simulink model "FullyConnectedMMG"  (R2020b)
settings: Solver=ode3  StartTime=0.0  StopTime=TimeS  FixedStep=Ts  RelTol=1e-3
values from neighbouring files (symbols this model uses):
  fr = 60    [MMG_Parameters.m]
  Lgs = 600e-6    (= 0.0006)    [MMG_Parameters.m]
  MaxWind = 18    [MMG_Parameters.m]
  MicroVol = 575    [MMG_Parameters.m]
  MinWind = 3    [MMG_Parameters.m]
  NomVol = 600    [MMG_Parameters.m]
  NomWind = 10    [MMG_Parameters.m]
  Pnombb = 400    [MMG_Parameters.m]
  PnomDG = 150e3    (= 150000)    [MMG_Parameters.m]
  PnomWT = 400e3    (= 400000)    [MMG_Parameters.m]
  Rgs = 20e-6    (= 2e-05)    [MMG_Parameters.m]
  RtCapM1 = (5.1)*1e-1    (= 0.51)    [MMG_Parameters.m]
  RtCapM2 = (5.1)*1e-1    (= 0.51)    [MMG_Parameters.m]
  SOC = [70,80,75,65]    [MMG_Parameters.m]
  Ts = 8e-4    (= 0.0008)    [MMG_Parameters.m]    (also in SolveMONO.m = 0.005)
  Vgrid = 25e3    (= 25000)    [MMG_Parameters.m]
  VMic = 575    [MMG_Parameters.m]
  Vs = 120e3    (= 120000)    [MMG_Parameters.m]
undefined symbols (not defined in the file or in its folder): DiscIntNeverNeededParam
libraries: powerlib x64, simulink x24, powerlib_meascontrol x16
(part 2 of 5)

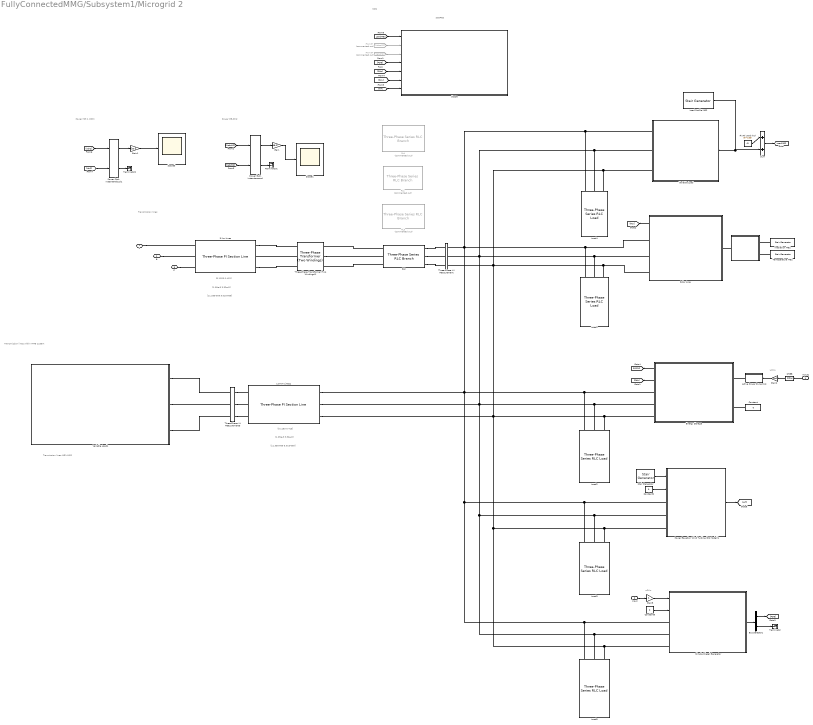
== system FullyConnectedMMG/Subsystem1/Microgrid 2 ==
  note: [0.1153 0.413]
  note: SCOPES
  note: w2Kw
  note: w2Kw
  note: MG2
  note: Transmission lines
  note: Power MG-Grid
  note: [0.1153 0.413]
  note: Transmission lines within MMG system
  note: [11.33e-009 5.01e-009]
  note: Tranmission lines MG1-MG2
  note: [1.05e-3 3.32e-3]
  note: [1.05e-3 3.32e-3]
  note: [11.33e-009 5.01e-009]
  note: Power MG 2 -MGm
  Input1 : Inport
  Input : Inport  Port=2
  " " : Subsystem  VariantControl=T6NotZero  mask{Pvr=200, Dfac=0.98, Tfac=0.3, Tsc=25}
      mask prompts: Pvr "Rated Power (kW)"; Dfac "Derating Factor"; Tfac "Temperature Factor"; Tsc "Standard Temperature (C)"
  1.5 Km Lines1 : powerlib/Elements/Three-Phase PI Section Line  LConnTagsString=a|b|c  RConnTagsString=A|B|C  Length=1.5  Frequency=fr  Resistances=[0.1153 1.413]  Inductances=[1.05e-3 3.32e-3]  Capacitances=[11.33e-009 5.01e-009]
  3 Km Lines : powerlib/Elements/Three-Phase PI Section Line  LConnTagsString=a|b|c  RConnTagsString=A|B|C  Length=3.5  Frequency=fr  Resistances=[0.0153 0.213]  Inductances=[1.05e-3 3.32e-3]  Capacitances=[11.33e-009 5.01e-009]
  Active Power Dynamics : Subsystem  VariantControl=T6NotZero
      mask Display: disp('1 / (1 + s T_P)','texmode','on');
  Bus Selector1 : BusSelector  OutputSignals=Active power P (W),Reactive power Q (var)
  Constant : Constant  Value=0
  Constant2 : Constant  Value=0
  Constant5 : Constant  Value=0
  Energy Storage : Subsystem  mask(Grid-connected Energy Storage (PQ Model)){Vn=NomVol, Fn=60, PnomkW=Pnombb, kWh_Rated=RtCapM2, Efficiency=96, LimitVec=[90 10], RechargeSOC=11, Precharge=50, autoRecharge=off, Initial_kWh_pc=SOC(2), PQvec=[500e3 0]}
      mask prompts: Vn "Nominal L-L Voltage [Vrms]"; Fn "Nominal Frequency [Hz]"; PnomkW "Rated Power [kW]"; kWh_Rated "Rated Capacity [kWh]"; Efficiency "Overall System Efficiency [%]"; LimitVec "Upper/Lower Charge Limits [%]"; RechargeSOC "SOC to Recharge [%]"; Precharge "Recharge Rate [% of Rated Power]"; autoRecharge "Enable Auto-Recharge"; Initial_kWh_pc "Initial State-of-Charge [0-100%]"; PQvec "Initial Active/Reactive Cmds"
      mask help:
      | The energy storage block models a generic grid-connected energy storage system (ESS), most commonly a battery system. This is a system-level model that does not contain any power electronics, but is useful for load flow, phasor, and hybrid phasor-EMT simulations. The inputs to this block are the commanded active and reactive power of the ESS. The ESS is assumed to have four quadrent operation.
      |
      | For more detailed ESS models, consider the battery block in the Drives library. Consider using this PQ Model to perform load flow studies and switch to a more detailed model when full EMT studies or more advanced controls are required.
      |
      | Note: The initial active/reactive power commands must be specified for use for Load Flow analysis.
      mask init: same as FullyConnectedMMG/Subsystem1/Microgrid 1/Energy Storage
      mask DialogControl Container7 Prompt: Grid Connection Properties
      mask DialogControl Container11 Prompt: Charge/Discharge Controls
      mask DialogControl Container12 Prompt: Initial Conditions
      mask Display: image(imread('Battery.png'))
  Fixed Load (Kw) : Constant  Value=(3)*(1e3)  VectorParams1D=off
  From34 : From  Commented=on  GotoTag=IabcM2  TagVisibility=global
      settings: CloseFcn=tagdialog Close
  From37 : From  Commented=on  GotoTag=VabcM2  TagVisibility=global
      settings: CloseFcn=tagdialog Close
  Gain : Gain  Gain=1e-3
  Gain1 : Gain  Gain=1e-3
  Gain2 : Gain  Gain=1e0
  Gain5 : Gain
  Irradiation MG2 : powerlib_meascontrol/Pulse & Signal Generators/Stair Generator  t=Time  e=IrMG2  Ts=Ts
  Load Profile MG2 : powerlib_meascontrol/Pulse & Signal Generators/Stair Generator  t=Time  e=PLoad2  Ts=Ts
  Load{1..5} (5 alike) : powerlib/Elements/Three-Phase Series RLC Load  LConnTagsString=A|B|C  Configuration=Y (grounded)  NominalVoltage=575  Vabc=[1e3 1e3 1e3]  Vabcp=[1e3 1e3 1e3]  NominalFrequency=60  UnbalancedPower=off  ActivePower=1e3  InductivePower=0  CapacitivePower=0  Pabc=[10e3 9e3 11e3]  QLabc=[100 90 110]  QCabc=[100 90 110]  Pabcp=[10e3 9e3 11e3]  QLabcp=[100 90 110]  QCabcp=[100 90 110]  Measurements=None  LoadType=constant Z
      settings: AttributesFormatString=P = %<ActivePower> W
  "Power (3ph, Instantaneous)" : powerlib_meascontrol/Measurements/Power (3ph, Instantaneous)
  "Power (3ph, Instantaneous)1" : powerlib_meascontrol/Measurements/Power (3ph, Instantaneous)
  Power Equation Wind Turbine (PQ Model)1 : Subsystem  AncestorBlock=|  mask{Unom=NomWind, Umax=MaxWind, Umin=MinWind, Pselect=Simple Cubic Power, rp=5, Cp=16/27, rho=1.225, Pnom=PnomWT, Uvec=[1:1:30], Pvec=1e-1*[0,0,0,0,21359.3750000000,58193.5000000000,104316.125000000,157104.500000000,213935.875000000,272187.500000000,329236.625000000,382460.500000000,429236.375000000,466941.500000000,492953.125000000,500000,500000,500000,500000,500000,500000,500000,500000,500000,500000,0,0,0,0,0], Tp=0.1, Tq=1, ReactP=30}
      | exampleMicrogridLibrary/Power Equation
      | Wind Turbine
      | (PQ Model)
      mask prompts: Unom "Nominal Wind Speed [m/s]"; Umax "Maximum Operating Wind [m/s]"; Umin "Minimum Operating Wind [m/s]"; Pselect "Wind Turbine Power Method"; rp "Blade Radius, r [m]"; Cp "Performance Coefficient, Cp"; rho "Air Density, rho [kg/m^3]"; Pnom "Nominal Power, [W]"; Uvec "Wind Vec [m/s]"; Pvec "Power Vec [W]"; Tp "Active Power Dynamics, Tp [s]"; Tq "Reactive Power Dynamics, Tq [s]"; ReactP "Reactive Power Percentage [%]"
      mask help:
      | Simple Wind Turbine that serves as an Active and Reactive Power Source depending on the Wind Power Curve.
      |
      | The Wind Turbine Power Curve can be defined by:
      | - Dimentions of the wind turbine
      | - Simple cubic power curve
      | - Look-up vector from a wind turbine data sheet.
      mask init:
      | A = pi*rp^2;
      | 
      | if Pselect == 1,
      |     Pmax = 1/2*rho*Cp*A*Umax^3;
      | elseif Pselect == 2,
      |     Pmax = Pnom;
      | else
      |     Pmax = max(Pvec);
      | end
      | Qmax = ReactP/100*Pmax;
      mask TypeOptions Pselect: Using Properties | Simple Cubic Power | Look-up Fit
      mask DialogControl Container4 Prompt: General
      mask DialogControl Container9 Prompt: Dimensions
      mask DialogControl Container12 Prompt: Cubic
      mask DialogControl Container7 Prompt: Lookup
      mask DialogControl Container8 Prompt: Dynamics
      mask Display:
      | image(imread('eolienne.bmp'))
      | 
      | color('white')
      | port_label('LConn',1,'A')
      | port_label('LConn',2,'B')
      | port_label('LConn',3,'C')
      | 
      | color('blue')
      | port_label('output',1,'m')
      | port_label('input',1,'Wind (m/s)')
      | port_label('input',2,'Qref')
  RL1 : powerlib/Elements/Three-Phase Series RLC Branch  Commented=on  LConnTagsString=A|B|C  RConnTagsString=A|B|C  BranchType=RL  Resistance=Rgs  Inductance=Lgs  Capacitance=inf  Measurements=None
  RL2 : powerlib/Elements/Three-Phase Series RLC Branch  LConnTagsString=A|B|C  RConnTagsString=A|B|C  BranchType=RL  Resistance=Rgs  Inductance=70e-6  Capacitance=inf  Measurements=None
  RL3 : powerlib/Elements/Three-Phase Series RLC Branch  Commented=on  LConnTagsString=A|B|C  RConnTagsString=A|B|C  BranchType=RL  Resistance=Rgs  Inductance=Lgs  Capacitance=inf  Measurements=None
  RL4 : powerlib/Elements/Three-Phase Series RLC Branch  Commented=on  LConnTagsString=A|B|C  RConnTagsString=A|B|C  BranchType=RL  Resistance=Rgs  Inductance=Lgs  Capacitance=inf  Measurements=None
  Scope : Subsystem
  Scope1 : Scope
  Scope3 : Scope
  Simple Diesel Generator : Subsystem  AncestorBlock=|  mask{Pn=PnomDG, Vn=VMic, Fn=fr, Tp=0.1, Tq=1, ReactP=30, Ts=Ts}
      | exampleMicrogridLibrary/Power Equation
      | Wind Turbine
      | (PQ Model)
      mask prompts: Pn "Generator Rated Power [W]"; Vn "Rated Voltage [V]"; Fn "Rated Frequency [Hz]"; Tp "Active Power Dynamics, Tp [s]"; Tq "Reactive Power Dynamics, Tq [s]"; ReactP "Reactive Power Percentage [%]"; Ts "Sample Time"
      mask help:
      | Simple Wind Turbine that serves as an Active and Reactive Power Source depending on the Wind Power Curve.
      |
      | The Wind Turbine Power Curve can be defined by:
      | - Dimentions of the wind turbine
      | - Simple cubic power curve
      | - Look-up vector from a wind turbine data sheet.
      mask init:
      | Pmax = 320e3;
      | Qmax = ReactP/100*Pmax;
      mask DialogControl Container4 Prompt: General
      mask DialogControl Container8 Prompt: Dynamics
      mask Display:
      | image(imread('DGEN.jpg'));
      | color('black')
  Solar Array : Subsystem  mask(Grid-Connected PV Array (PQ Model)){Vn=MicroVol, Fn=fr, P0=500e3}
      mask prompts: Vn "Nominal L-L Voltage [Vrms]"; Fn "Nominal Frequency [Hz]"; P0 "Initial Power [W]"
      mask help:
      | This block models a grid-connected solar array using the Three-Phase Dynamic Load block. This is a system-level model that does not contain any power electronics, but is useful for load flow, phasor, and hybrid phasor-EMT simulations. The input to this block is the power output of the grid connected PV array, not irradiance.
      |
      | For more detailed PV models, consider the PV Array block in the Renewables library. Consider using this PQ Model to perform load flow studies and switch to a more detailed model when full EMT studies are required.
      |
      | Note: The array power must be specified for use for Load Flow analysis.
      mask init:
      | % P0 = Irr0*TotalArea*Efficiency/100;
      | P0 = -P0;
      mask Display:
      | image(imread('PV_Farm.jpg'))
      | color('white')
      | port_label('input',1,'P')
      | port_label('output',1,'m')
      | port_label('Rconn',1,'A')
      | port_label('Rconn',2,'B')
      | port_label('Rconn',3,'C')
  Stair Generator : powerlib_meascontrol/Pulse & Signal Generators/Stair Generator  t=Time  e=WindM2  Ts=Ts
  Sum : Sum  Inputs=|++
  Temeperature MG2 : powerlib_meascontrol/Pulse & Signal Generators/Stair Generator  t=Time  e=TempMG2  Ts=Ts
  Terminator : Terminator
  Terminator1 : Terminator
  Terminator2 : Terminator
  Three-Phase Transformer (Two Windings)1 : powerlib/Elements/Three-Phase Transformer (Two Windings)  Winding1Connection=Yg  Winding2Connection=Yg  CoreType=Three single-phase transformers  SetSaturation=off  Hysteresis=off  DataFile='hysteresis'  SetInitialFlux=off  Measurements=None  UNITS=pu  NominalPower=[ 25e6 , 60 ]  Winding1=[575 , 0.002 , 0.08 ]  Winding2=[575 , 0.002 , 0.08 ]  Rm=500  Lm=500  L0=0.5  Saturation=[ 0,0 ; 0.0024,1.2 ; 1.0,1.52 ]  InitialFluxes=[ 0.8 , -0.8 , 0.7 ]  BreakLoop=off  DiscreteSolver=Trapezoidal iterative  DataType=off  TransfoNumber=1
  Three-Phase V-I Measurement : powerlib/Measurements/Three-Phase V-I Measurement  VoltageMeasurement=phase-to-ground  SetLabelV=on  LabelV=VabcM2  Vpu=off  VpuLL=off  CurrentMeasurement=yes  SetLabelI=on  LabelI=IabcM2  Ipu=off  Pbase=100e6  Vbase=500e3  OutputType=Complex  PhasorSimulation=off  PSBequivalent=0
  Three-Phase V-I Measurement3 : powerlib/Measurements/Three-Phase V-I Measurement  VoltageMeasurement=phase-to-ground  SetLabelV=on  LabelV=Vsh2  Vpu=off  VpuLL=off  CurrentMeasurement=yes  SetLabelI=on  LabelI=Ish2  Ipu=off  Pbase=100e6  Vbase=500e3  OutputType=Complex  PhasorSimulation=off  PSBequivalent=0
  Variable Load : Subsystem  mask(Variable Load (PQ Model)){Vn=MicroVol, Fn=fr, PF=1, Load0=20e3}
      mask prompts: Vn "Nominal L-L Voltage [Vrms]"; Fn "Nominal Frequency [Hz]"; PF "Power Factor [0 to 1]"; Load0 "Initial Load [W]"
      mask help:
      | The Variable Load block is a lumped approximation for a distribution feeder. For non-unity power factor loads, the input (active power) is scaled accordingly to generate a desired load.
      |
      | Note: The initial input load must be specified for use for Load Flow analysis.
      mask init:
      | P0 = Load0;
      | Q0 = Load0*sqrt(1/PF-1);
      mask Display:
      | image(imread('Residential.jpg'))
      | color('white')
      | port_label('input',1,'Load')
      | port_label('Rconn',1,'A')
      | port_label('Rconn',2,'B')
      | port_label('Rconn',3,'C')
  Variable Load1 : Subsystem  mask(Variable Load (PQ Model)){Vn=MicroVol, Fn=fr, PF=1, Load0=20e3}
      mask prompts: Vn "Nominal L-L Voltage [Vrms]"; Fn "Nominal Frequency [Hz]"; PF "Power Factor [0 to 1]"; Load0 "Initial Load [W]"
      mask help:
      | The Variable Load block is a lumped approximation for a distribution feeder. For non-unity power factor loads, the input (active power) is scaled accordingly to generate a desired load.
      |
      | Note: The initial input load must be specified for use for Load Flow analysis.
      mask init:
      | P0 = Load0;
      | Q0 = Load0*sqrt(1/PF-1);
      mask Display:
      | image(imread('Sharing.jpg'))
      | color('black')
      | % port_label('input',1,'Load')
      | port_label('Rconn',1,'A')
      | port_label('Rconn',2,'B')
      | port_label('Rconn',3,'C')
  ZHBB : ZeroOrderHold  SampleTime=Ts
  A : PMIOPort  Side=Left
  B : PMIOPort  Port=2  Side=Left
  C : PMIOPort  Port=3  Side=Left
  tag scope: LoadMG2=global, SOCM2=global
  wires:
  Sum/1 -> [LoadMG2]
  Solar Array/1(m) -> [Ppv]
  Load Profile MG2/1 -> Sum/2, Variable Load/1(Load)
  Fixed Load (Kw)/1 -> Sum/1
  Power Equation Wind Turbine (PQ Model)1/1(m) -> [WT]
  Constant2/1 -> Power Equation Wind Turbine (PQ Model)1/2(Qref (pu))
  Gain2/1 -> Active Power Dynamics/1(In)
  " "/1(PowerOut) -> Solar Array/1(P)
  Gain5/1 -> Simple Diesel Generator/1(Pref (pu))
  Bus Selector1/1 -> [PDG]  "<Active power P (W)>"
  Bus Selector1/2 -> Terminator/1  "<Reactive power Q (var)>"
  Constant5/1 -> Simple Diesel Generator/2(Qref (pu))
  Simple Diesel Generator/1(m) -> Bus Selector1/1
  Input1/1 -> ZHBB/1
  ZHBB/1 -> Gain2/1
  Input/1 -> Gain5/1
  Stair Generator/1 -> Power Equation Wind Turbine (PQ Model)1/1(Wind (m/s))
  Irradiation MG2/1 -> " "/1(Irra)
  Temeperature MG2/1 -> " "/2(Temp)
  Energy Storage/2(Pbatt) -> [Pbb]
  Constant/1 -> Energy Storage/2(Qref)
  Active Power Dynamics/1(Out) -> Energy Storage/1(Pref)
  [LoadMG2] -> Scope/1(LOAD)  "Load M2"
  From37/1 -> Scope/2(VABC)
  From34/1 -> Scope/3(IABC)
  [PDG] -> Scope/4(PDG)
  [Pbb] -> Scope/5(PBB)
  [Ppv] -> Scope/6(PPV)
  [WT] -> Scope/7(PWT)
  Energy Storage/1(SOC (%)) -> [SOCM2]
  [VabcM2] -> "Power (3ph, Instantaneous)"/1
  "Power (3ph, Instantaneous)"/2 -> Terminator1/1
  Gain/1 -> Scope1/1
  "Power (3ph, Instantaneous)"/1 -> Gain/1
  [IabcM2] -> "Power (3ph, Instantaneous)"/2
  "Power (3ph, Instantaneous)1"/1 -> Gain1/1
  [Ish2] -> "Power (3ph, Instantaneous)1"/2
  "Power (3ph, Instantaneous)1"/2 -> Terminator2/1
  Gain1/1 -> Scope3/1
  [Vsh2] -> "Power (3ph, Instantaneous)1"/1
  connections:
  Three-Phase Transformer (Two Windings)1/LConn2 -- 3 Km Lines/LConn2
  3 Km Lines/LConn1 -- Three-Phase Transformer (Two Windings)1/LConn1
  3 Km Lines/LConn3 -- Three-Phase Transformer (Two Windings)1/LConn3
  A/RConn1 -- 3 Km Lines/RConn1
  B/RConn1 -- 3 Km Lines/RConn2
  C/RConn1 -- 3 Km Lines/RConn3
  RL2/RConn1 -- Three-Phase Transformer (Two Windings)1/RConn1
  RL2/RConn3 -- Three-Phase Transformer (Two Windings)1/RConn3
  Three-Phase Transformer (Two Windings)1/RConn2 -- RL2/RConn2
  Variable Load/RConn1 -- Load4/LConn1 -- 1.5 Km Lines1/LConn1 -- Load5/LConn1 -- Simple Diesel Generator/LConn1 -- Load3/LConn1 -- Power Equation Wind Turbine (PQ Model)1/LConn1 -- Energy Storage/RConn1 -- Load2/LConn1 -- Solar Array/RConn1 -- Load1/LConn1 -- Three-Phase V-I Measurement/RConn1
  Variable Load/RConn2 -- Load4/LConn2 -- 1.5 Km Lines1/LConn2 -- Load5/LConn2 -- Simple Diesel Generator/LConn2 -- Load3/LConn2 -- Power Equation Wind Turbine (PQ Model)1/LConn2 -- Energy Storage/RConn2 -- Load2/LConn2 -- Load1/LConn2 -- Solar Array/RConn2 -- Three-Phase V-I Measurement/RConn2
  Variable Load/RConn3 -- Load4/LConn3 -- 1.5 Km Lines1/LConn3 -- Load5/LConn3 -- Simple Diesel Generator/LConn3 -- Load3/LConn3 -- Power Equation Wind Turbine (PQ Model)1/LConn3 -- Energy Storage/RConn3 -- Load2/LConn3 -- Load1/LConn3 -- Solar Array/RConn3 -- Three-Phase V-I Measurement/RConn3
  Variable Load1/RConn3 -- Three-Phase V-I Measurement3/RConn3
  Variable Load1/RConn1 -- Three-Phase V-I Measurement3/RConn1
  Variable Load1/RConn2 -- Three-Phase V-I Measurement3/RConn2
  Three-Phase V-I Measurement3/LConn1 -- 1.5 Km Lines1/RConn1
  Three-Phase V-I Measurement3/LConn2 -- 1.5 Km Lines1/RConn2
  Three-Phase V-I Measurement3/LConn3 -- 1.5 Km Lines1/RConn3
  RL2/LConn2 -- Three-Phase V-I Measurement/LConn2
  RL2/LConn1 -- Three-Phase V-I Measurement/LConn1
  RL2/LConn3 -- Three-Phase V-I Measurement/LConn3

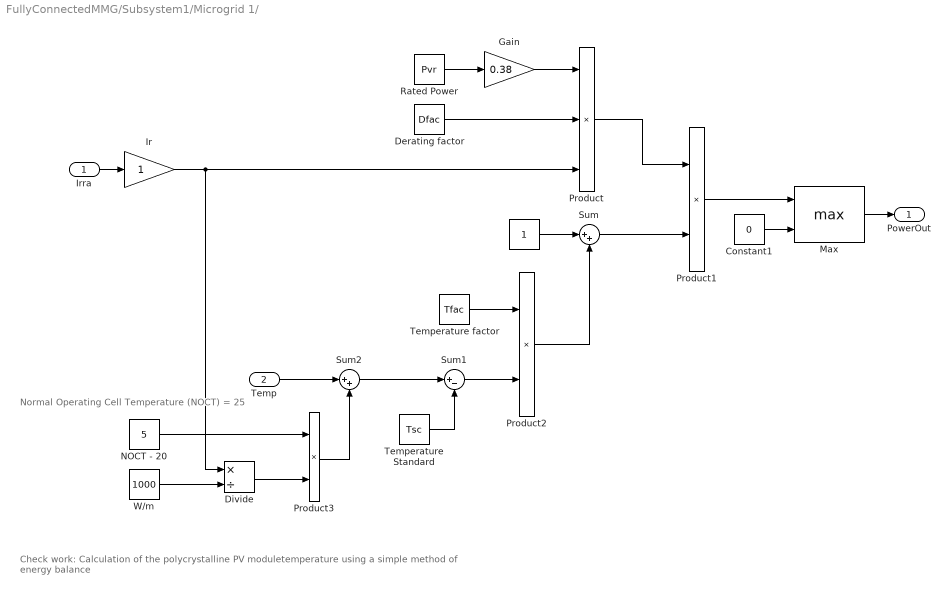
== system FullyConnectedMMG/Subsystem1/Microgrid 1/  ==
  note: Check work: Calculation of the polycrystalline PV moduletemperature using a simple method of energy balance
  note: Normal Operating Cell Temperature (NOCT) = 25
  Irra : Inport
  Temp : Inport  Port=2
  " " : Constant
  Constant1 : Constant  Value=0
  Derating factor : Constant  Value=Dfac
  Divide : Product  Inputs=*/
  Gain : Gain  Gain=0.38
  Ir : Gain
  Max : MinMax  Function=max  Inputs=2
  NOCT - 20 : Constant  Value=5
  Product : Product  Inputs=3
  Product1 : Product
  Product2 : Product
  Product3 : Product
  Rated Power : Constant  Value=Pvr
  Sum : Sum  Inputs=|++
  Sum1 : Sum  Inputs=|+-
  Sum2 : Sum  Inputs=|++
  Temperature Standard : Constant  Value=Tsc
  Temperature factor : Constant  Value=Tfac
  W/m : Constant  Value=1000
  PowerOut : Outport  VectorParamsAs1DForOutWhenUnconnected=off
  wires:
  Rated Power/1 -> Gain/1
  Gain/1 -> Product/1
  Derating factor/1 -> Product/2
  Irra/1 -> Ir/1
  Product/1 -> Product1/1
  " "/1 -> Sum/1
  Product2/1 -> Sum/2
  Temperature factor/1 -> Product2/1
  Sum/1 -> Product1/2
  Sum1/1 -> Product2/2
  Temperature Standard/1 -> Sum1/2
  Temp/1 -> Sum2/1
  Sum2/1 -> Sum1/1
  Product3/1 -> Sum2/2
  NOCT - 20/1 -> Product3/1
  Divide/1 -> Product3/2
  W/m/1 -> Divide/2
  Ir/1 -> Divide/1, Product/3
  Constant1/1 -> Max/2
  Max/1 -> PowerOut/1
  Product1/1 -> Max/1

== system FullyConnectedMMG/Subsystem1/Microgrid 1/Active Power Dynamics1 ==
  In : Inport
  1/Tp : Gain  Gain=1/0.004
  Integrator : Integrator
  Sum : Sum  Inputs=|+-
  Out : Outport  VectorParamsAs1DForOutWhenUnconnected=off
  wires:
  Integrator/1 -> Out/1, Sum/2
  In/1 -> Sum/1
  1/Tp/1 -> Integrator/1
  Sum/1 -> 1/Tp/1

== system FullyConnectedMMG/Subsystem1/Microgrid 1/Energy Storage ==
  Pref : Inport
  Qref : Inport  Port=2
  Charge Limits : Subsystem
  Mux1 : Mux  Inputs=2
  Power Limits : Saturate  UpperLimit=Pnom  LowerLimit=-Pnom
  Reactive Power Capability : Subsystem
  Simple Battery Inverter : powerlib/Elements/Three-Phase Dynamic Load  NominalVoltage=[Vn Fn]  ActiveReactivePowers=[-500000 -3.38813e-13]  PositiveSequence=[0.999844 -0.0038635]  ExternalControl=on  NpNq=[1.3 2]  TimeConstants="[0  0  0  0]"  MinimumVoltage=0.7  Tfilter=1e-2  LoadFlowParameters=[4,0,0,0,0]
      link override Model/Discrete 3-phase PLL: Ts=Ts
      link override Model/Mean (Variable Frequency): Ts=Ts
      link override Model/Mean (Variable Frequency)1: Ts=Ts
      settings: SourceProductBaseCode=PS
  Stored Energy Calculation (%) : Subsystem
  Terminator : Terminator
  Unary Minus : UnaryMinus
  A : PMIOPort  Side=Right
  B : PMIOPort  Port=2  Side=Right
  C : PMIOPort  Port=3  Side=Right
  SOC (%) : Outport  VectorParamsAs1DForOutWhenUnconnected=off
  Pbatt : Outport  Port=2  VectorParamsAs1DForOutWhenUnconnected=off
  wires:
  Charge Limits/2(Qbatt) -> Reactive Power Capability/2(Qin)
  Qref/1 -> Charge Limits/3(Qin)
  Power Limits/1 -> Charge Limits/2(Pin)
  Charge Limits/1(Pbatt) -> Reactive Power Capability/1(Pin), Unary Minus/1, Pbatt/1, Stored Energy Calculation (%)/1(Pin)  "Pbatt"
  Stored Energy Calculation (%)/1(SE%) -> SOC (%)/1, Charge Limits/1(SOC (%))  "SOC (%)"
  Pref/1 -> Power Limits/1
  Reactive Power Capability/1(Qout) -> Mux1/2, Stored Energy Calculation (%)/2(Qin)  "Qbatt"
  Simple Battery Inverter/1 -> Terminator/1
  Mux1/1 -> Simple Battery Inverter/1
  Unary Minus/1 -> Mux1/1
  connections:
  Simple Battery Inverter/LConn1 -- A/RConn1
  Simple Battery Inverter/LConn3 -- C/RConn1
  Simple Battery Inverter/LConn2 -- B/RConn1

== system FullyConnectedMMG/Subsystem1/Microgrid 1/Power Equation Wind Turbine (PQ Model) ==
  Wind (m/s) : Inport
  Qref (pu) : Inport  Port=2
  Active Power Dynamics : Subsystem  VariantControl=T6NotZero
      mask Display: disp('1 / (1 + s T_P)','texmode','on');
  Ground : powerlib/Elements/Ground  LConnTagsString=a
  Mux : Mux  Inputs=2
  Reactive Power Dynamics : Subsystem  VariantControl=T6NotZero
      mask Display: disp('1 / (1 + s T_Q)','texmode','on');
  Saturation : Saturate  UpperLimit=Qmax  LowerLimit=-Qmax
  Scope : Scope
  Shunt (Numerical Stability) : powerlib/Elements/Three-Phase Series RLC Branch  LConnTagsString=A|B|C  RConnTagsString=A|B|C  BranchType=R  Resistance=1e3  Inductance=1e-3  Capacitance=1e-6  Measurements=None
  Three-Phase Dynamic Load : powerlib/Elements/Three-Phase Dynamic Load  NominalVoltage=[575 60]  ActiveReactivePowers=[20e3 1e3]  PositiveSequence=[0.994 -11.8]  ExternalControl=on  NpNq=[1.3 2]  TimeConstants="[0  0  0  0]"  MinimumVoltage=0.7  Tfilter=1e-4  LoadFlowParameters=[4,0,0,0,0]
      link override Model/Discrete 3-phase PLL: Ts=Ts
      link override Model/Mean (Variable Frequency): Ts=Ts
      link override Model/Mean (Variable Frequency)1: Ts=Ts
      settings: SourceProductBaseCode=PS
  Unary Minus : UnaryMinus
  Wind Turbine Power Equation : Subsystem
  A : PMIOPort  Side=Left
  B : PMIOPort  Port=2  Side=Left
  C : PMIOPort  Port=3  Side=Left
  m : Outport  VectorParamsAs1DForOutWhenUnconnected=off
  wires:
  Qref (pu)/1 -> Saturation/1
  Saturation/1 -> Reactive Power Dynamics/1(In)
  Reactive Power Dynamics/1(Out) -> Mux/2
  Mux/1 -> Three-Phase Dynamic Load/1
  Wind Turbine Power Equation/1(Pwind) -> Active Power Dynamics/1(In)
  Wind (m/s)/1 -> Wind Turbine Power Equation/1(Wind (m/s))
  Three-Phase Dynamic Load/1 -> m/1
  Active Power Dynamics/1(Out) -> Unary Minus/1
  Unary Minus/1 -> Scope/1, Mux/1
  connections:
  Ground/LConn1 -- Shunt (Numerical Stability)/RConn1 -- Shunt (Numerical Stability)/RConn2 -- Shunt (Numerical Stability)/RConn3
  Three-Phase Dynamic Load/LConn1 -- Shunt (Numerical Stability)/LConn1 -- A/RConn1
  Three-Phase Dynamic Load/LConn3 -- Shunt (Numerical Stability)/LConn3 -- C/RConn1
  Three-Phase Dynamic Load/LConn2 -- Shunt (Numerical Stability)/LConn2 -- B/RConn1

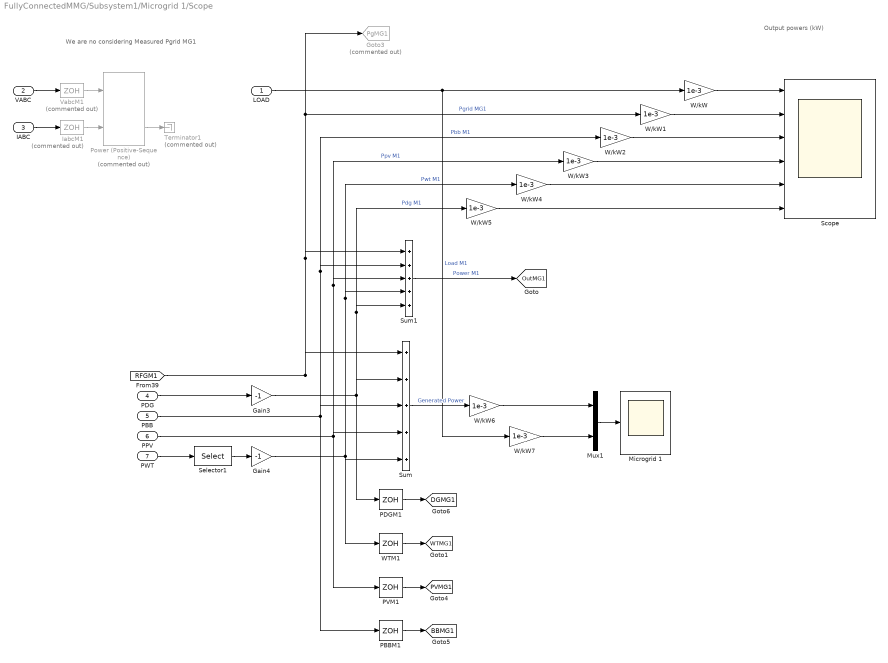
== system FullyConnectedMMG/Subsystem1/Microgrid 1/Scope ==
  note: Output powers (kW)
  note: We are no considering Measured Pgrid MG1
  LOAD : Inport
  VABC : Inport  Port=2
  IABC : Inport  Port=3
  PDG : Inport  Port=4
  PBB : Inport  Port=5
  PPV : Inport  Port=6
  PWT : Inport  Port=7
  Gain3 : Gain  Gain=-1
  Gain4 : Gain  Gain=-1
  Goto3 : Goto  Commented=on  GotoTag=PgMG1  TagVisibility=global
  IabcM1 : ZeroOrderHold  Commented=on  SampleTime=Ts
  Microgrid 1 : Scope
  Mux1 : Mux  Inputs=2
  PBBM1 : ZeroOrderHold  SampleTime=Ts
  PDGM1 : ZeroOrderHold  SampleTime=Ts
  PVM1 : ZeroOrderHold  SampleTime=Ts
  Power (Positive-Sequence) : powerlib_meascontrol/Measurements/Power (Positive-Sequence)  Commented=on  Freq=60  Vinit=[0, 0]  Iinit=[0, 0]  Ts=3e-4
      settings: SourceProductBaseCode=PS
  Scope : Scope  NumInputPorts=6
  Selector1 : Selector  InputPortWidth=3  IndexOptions=Index vector (dialog)  Indices=[2]  OutputSizes=1
  Sum : Sum  Inputs=|+++++
  Sum1 : Sum  Inputs=|+++++
  Terminator1 : Terminator  Commented=on
  VabcM1 : ZeroOrderHold  Commented=on  SampleTime=Ts
  W/kW{,1..7} (8 alike) : Gain  Gain=1e-3
  WTM1 : ZeroOrderHold  SampleTime=Ts
  tag scope: BBMG1=global, DGMG1=global, OutMG1=global, PVMG1=global, WTMG1=global
  wires:
  Power (Positive-Sequence)/2 -> Terminator1/1
  PPV/1 -> Sum/4, PVM1/1, Sum1/3, W/kW3/1  "Ppv M1"
  PBB/1 -> PBBM1/1, Sum/3, Sum1/2, W/kW2/1  "Pbb M1"
  [RFGM1] -> Sum1/1, Goto3/1, W/kW1/1, Sum/1  "Pgrid MG1"
  Mux1/1 -> Microgrid 1/1
  LOAD/1 -> W/kW7/1, W/kW/1  "Load M1"
  Gain4/1 -> WTM1/1, Sum/5, Sum1/4, W/kW4/1  "Pwt M1"
  PWT/1 -> Selector1/1
  Selector1/1 -> Gain4/1
  Sum1/1 -> [OutMG1]  "Power M1"
  Sum/1 -> W/kW6/1  "Generated Power"
  Gain3/1 -> PDGM1/1, Sum1/5, W/kW5/1, Sum/2  "Pdg M1"
  PDG/1 -> Gain3/1
  PDGM1/1 -> [DGMG1]
  PBBM1/1 -> [BBMG1]
  PVM1/1 -> [PVMG1]
  WTM1/1 -> [WTMG1]
  VabcM1/1 -> Power (Positive-Sequence)/1
  VABC/1 -> VabcM1/1
  IabcM1/1 -> Power (Positive-Sequence)/2
  IABC/1 -> IabcM1/1
  W/kW/1 -> Scope/1
  W/kW1/1 -> Scope/2
  W/kW2/1 -> Scope/3
  W/kW3/1 -> Scope/4
  W/kW4/1 -> Scope/5
  W/kW5/1 -> Scope/6
  W/kW6/1 -> Mux1/1
  W/kW7/1 -> Mux1/2

== system FullyConnectedMMG/Subsystem1/Microgrid 1/Simple Diesel Generator ==
  Pref (pu) : Inport
  Qref (pu) : Inport  Port=2
  Active Power Dynamics : Subsystem  VariantControl=T6NotZero
      mask Display: disp('1 / (1 + s T_P)','texmode','on');
  Ground : powerlib/Elements/Ground  LConnTagsString=a
  Mux : Mux  Inputs=2
  Reactive Power Dynamics : Subsystem  VariantControl=T6NotZero
      mask Display: disp('1 / (1 + s T_Q)','texmode','on');
  Saturation : Saturate  UpperLimit=Qmax  LowerLimit=-Qmax
  Shunt (Numerical Stability) : powerlib/Elements/Three-Phase Series RLC Branch  LConnTagsString=A|B|C  RConnTagsString=A|B|C  BranchType=R  Resistance=1e3  Inductance=1e-3  Capacitance=1e-6  Measurements=None
  Three-Phase Dynamic Load : powerlib/Elements/Three-Phase Dynamic Load  NominalVoltage=[Vn Fn]  ActiveReactivePowers=[20e3 1e3]  PositiveSequence=[0.994 -11.8]  ExternalControl=on  NpNq=[1.3 2]  TimeConstants="[0  0  0  0]"  MinimumVoltage=0.7  Tfilter=1e-4  LoadFlowParameters=[4,0,0,0,0]
      link override Model/Discrete 3-phase PLL: Ts=Ts
      link override Model/Discrete 3-phase PLL/Discrete PI Controller: Ts=Ts
      link override Model/Discrete 3-phase PLL/Discrete Rate Limiter: Ts=Ts
      link override Model/Discrete 3-phase PLL/Discrete Variable Frequency Mean value: Ts=Ts
      link override Model/Mean (Variable Frequency): Ts=Ts
      link override Model/Mean (Variable Frequency)1: Ts=Ts
      settings: SourceProductBaseCode=PS
  Unary Minus : UnaryMinus
  A : PMIOPort  Side=Left
  B : PMIOPort  Port=2  Side=Left
  C : PMIOPort  Port=3  Side=Left
  m : Outport  VectorParamsAs1DForOutWhenUnconnected=off
  wires:
  Pref (pu)/1 -> Active Power Dynamics/1(In)
  Mux/1 -> Three-Phase Dynamic Load/1
  Reactive Power Dynamics/1(Out) -> Mux/2
  Saturation/1 -> Reactive Power Dynamics/1(In)
  Qref (pu)/1 -> Saturation/1
  Three-Phase Dynamic Load/1 -> m/1
  Active Power Dynamics/1(Out) -> Unary Minus/1
  Unary Minus/1 -> Mux/1
  connections:
  B/RConn1 -- Shunt (Numerical Stability)/LConn2 -- Three-Phase Dynamic Load/LConn2
  C/RConn1 -- Shunt (Numerical Stability)/LConn3 -- Three-Phase Dynamic Load/LConn3
  A/RConn1 -- Shunt (Numerical Stability)/LConn1 -- Three-Phase Dynamic Load/LConn1
  Shunt (Numerical Stability)/RConn3 -- Shunt (Numerical Stability)/RConn2 -- Shunt (Numerical Stability)/RConn1 -- Ground/LConn1

== system FullyConnectedMMG/Subsystem1/Microgrid 1/Solar Array ==
  P : Inport
  Active Power Dynamics : Subsystem  VariantControl=T6NotZero
      mask Display: disp('1 / (1 + s T_P)','texmode','on');
  Bus Selector : BusSelector  OutputSignals=Active power P (W)
  Constant11 : Constant  Value=0
  Mux1 : Mux  Inputs=2
  Simple Solar Inverter : powerlib/Elements/Three-Phase Dynamic Load  NominalVoltage=[Vn Fn]  ActiveReactivePowers=[-250000 -3.38813e-13]  PositiveSequence=[0.999844 -0.0038635]  ExternalControl=on  NpNq=[1.3 2]  TimeConstants="[0  0  0  0]"  MinimumVoltage=0.7  Tfilter=1e-2  LoadFlowParameters=[4,0,0,0,0]
      link override Model/Discrete 3-phase PLL/Discrete PI Controller: Ts=Ts
      link override Model/Discrete 3-phase PLL/Discrete Rate Limiter: Ts=Ts
      link override Model/Discrete 3-phase PLL/Discrete Variable Frequency Mean value: Ts=Ts
      settings: SourceProductBaseCode=PS
  Unary Minus : UnaryMinus
  Unary Minus1 : UnaryMinus
  A : PMIOPort  Side=Right
  B : PMIOPort  Port=2  Side=Right
  C : PMIOPort  Port=3  Side=Right
  m : Outport  VectorParamsAs1DForOutWhenUnconnected=off
  wires:
  P/1 -> Active Power Dynamics/1(In)
  Unary Minus/1 -> Mux1/1
  Mux1/1 -> Simple Solar Inverter/1
  Constant11/1 -> Mux1/2
  Simple Solar Inverter/1 -> Bus Selector/1
  Bus Selector/1 -> Unary Minus1/1  "<Active power P (W)>"
  Unary Minus1/1 -> m/1
  Active Power Dynamics/1(Out) -> Unary Minus/1
  connections:
  Simple Solar Inverter/LConn2 -- B/RConn1
  Simple Solar Inverter/LConn3 -- C/RConn1
  Simple Solar Inverter/LConn1 -- A/RConn1

== system FullyConnectedMMG/Subsystem1/Microgrid 1/Variable Load ==
  Load : Inport
  Active Power Dynamics : Subsystem  VariantControl=T6NotZero
      mask Display: disp('1 / (1 + s T_P)','texmode','on');
  Dynamic Load Control : Subsystem
  Simple Three-Phase Load : powerlib/Elements/Three-Phase Dynamic Load  NominalVoltage=[Vn Fn]  ActiveReactivePowers=[200000 45883.1]  PositiveSequence=[0.999844 -0.0038635]  ExternalControl=on  NpNq=[1.3 2]  TimeConstants="[0  0  0  0]"  MinimumVoltage=0.7  Tfilter=1e-2  LoadFlowParameters=[4,0,0,0,0]
      link override Model/Discrete 3-phase PLL: Ts=Ts
      link override Model/Discrete 3-phase PLL/Discrete PI Controller: Ts=Ts
      link override Model/Discrete 3-phase PLL/Discrete Rate Limiter: Ts=Ts
      link override Model/Discrete 3-phase PLL/Discrete Variable Frequency Mean value: Ts=Ts
      link override Model/Discrete 3-phase PLL/Discrete  2nd-Order Filter: Ts=Ts
      link override Model/Mean (Variable Frequency): Ts=Ts
      link override Model/Mean (Variable Frequency)1: Ts=Ts
      settings: SourceProductBaseCode=PS
  Terminator : Terminator
  A : PMIOPort  Side=Right
  B : PMIOPort  Port=2  Side=Right
  C : PMIOPort  Port=3  Side=Right
  wires:
  Simple Three-Phase Load/1 -> Terminator/1
  Dynamic Load Control/1(PQ) -> Simple Three-Phase Load/1
  Load/1 -> Active Power Dynamics/1(In)
  Active Power Dynamics/1(Out) -> Dynamic Load Control/1(P0)
  connections:
  Simple Three-Phase Load/LConn1 -- A/RConn1
  Simple Three-Phase Load/LConn3 -- C/RConn1
  Simple Three-Phase Load/LConn2 -- B/RConn1

== system FullyConnectedMMG/Subsystem1/Microgrid 1/Variable Load1 ==
  Active Power Dynamics : Subsystem  VariantControl=T6NotZero
      mask Display: disp('1 / (1 + s T_P)','texmode','on');
  Dynamic Load Control : Subsystem
  Load2 : powerlib/Elements/Three-Phase Series RLC Load  LConnTagsString=A|B|C  Configuration=Y (grounded)  NominalVoltage=575  Vabc=[1e3 1e3 1e3]  Vabcp=[1e3 1e3 1e3]  NominalFrequency=60  UnbalancedPower=off  ActivePower=1e3  InductivePower=0  CapacitivePower=0  Pabc=[10e3 9e3 11e3]  QLabc=[100 90 110]  QCabc=[100 90 110]  Pabcp=[10e3 9e3 11e3]  QLabcp=[100 90 110]  QCabcp=[100 90 110]  Measurements=None  LoadType=constant Z
      settings: AttributesFormatString=P = %<ActivePower> W
  Simple Three-Phase Load : powerlib/Elements/Three-Phase Dynamic Load  NominalVoltage=[Vn Fn]  ActiveReactivePowers=[200000 45883.1]  PositiveSequence=[0.999844 -0.0038635]  ExternalControl=on  NpNq=[1.3 2]  TimeConstants="[0  0  0  0]"  MinimumVoltage=0.7  Tfilter=1e-2  LoadFlowParameters=[4,0,0,0,0]
      link override Model/Discrete 3-phase PLL: Ts=Ts
      link override Model/Discrete 3-phase PLL/Discrete PI Controller: Ts=Ts
      link override Model/Discrete 3-phase PLL/Discrete Rate Limiter: Ts=Ts
      link override Model/Discrete 3-phase PLL/Discrete Variable Frequency Mean value: Ts=Ts
      link override Model/Discrete 3-phase PLL/Discrete  2nd-Order Filter: Ts=Ts
      link override Model/Mean (Variable Frequency): Ts=Ts
      link override Model/Mean (Variable Frequency)1: Ts=Ts
      settings: SourceProductBaseCode=PS
  Sum1 : Sum  Inputs=|++
  Terminator : Terminator
  A : PMIOPort  Side=Right
  B : PMIOPort  Port=2  Side=Right
  C : PMIOPort  Port=3  Side=Right
  wires:
  Simple Three-Phase Load/1 -> Terminator/1
  Dynamic Load Control/1(PQ) -> Simple Three-Phase Load/1
  Sum1/1 -> Active Power Dynamics/1(In)
  Active Power Dynamics/1(Out) -> Dynamic Load Control/1(P0)
  [rePM1] -> Sum1/2
  [shPM1] -> Sum1/1
  connections:
  Simple Three-Phase Load/LConn1 -- A/RConn1 -- Load2/LConn1
  Simple Three-Phase Load/LConn3 -- Load2/LConn3 -- C/RConn1
  Simple Three-Phase Load/LConn2 -- Load2/LConn2 -- B/RConn1

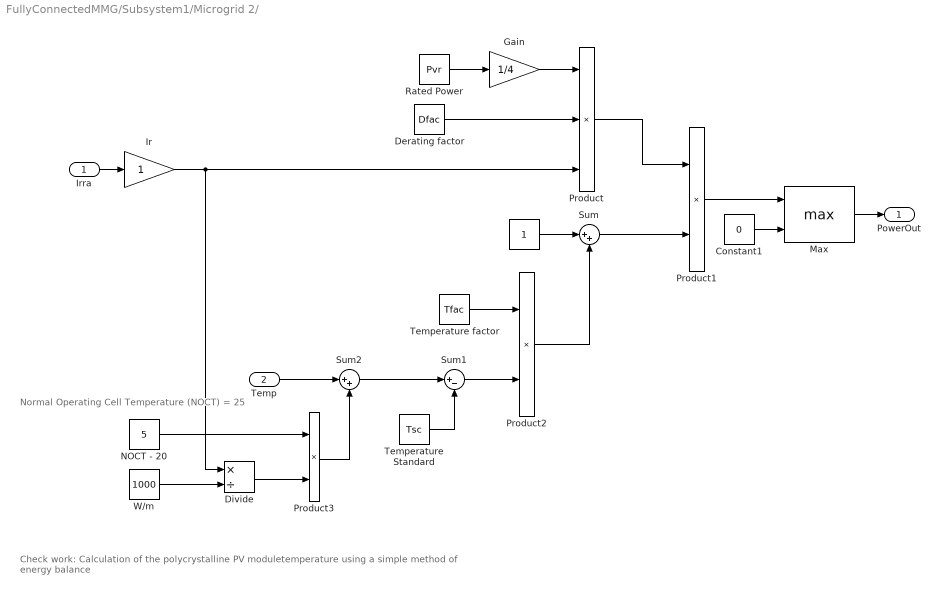
== system FullyConnectedMMG/Subsystem1/Microgrid 2/  ==
  note: Check work: Calculation of the polycrystalline PV moduletemperature using a simple method of energy balance
  note: Normal Operating Cell Temperature (NOCT) = 25
  Irra : Inport
  Temp : Inport  Port=2
  " " : Constant
  Constant1 : Constant  Value=0
  Derating factor : Constant  Value=Dfac
  Divide : Product  Inputs=*/
  Gain : Gain  Gain=1/4
  Ir : Gain
  Max : MinMax  Function=max  Inputs=2
  NOCT - 20 : Constant  Value=5
  Product : Product  Inputs=3
  Product1 : Product
  Product2 : Product
  Product3 : Product
  Rated Power : Constant  Value=Pvr
  Sum : Sum  Inputs=|++
  Sum1 : Sum  Inputs=|+-
  Sum2 : Sum  Inputs=|++
  Temperature Standard : Constant  Value=Tsc
  Temperature factor : Constant  Value=Tfac
  W/m : Constant  Value=1000
  PowerOut : Outport  VectorParamsAs1DForOutWhenUnconnected=off
  wires:
  Rated Power/1 -> Gain/1
  Gain/1 -> Product/1
  Derating factor/1 -> Product/2
  Irra/1 -> Ir/1
  Product/1 -> Product1/1
  " "/1 -> Sum/1
  Product2/1 -> Sum/2
  Temperature factor/1 -> Product2/1
  Sum/1 -> Product1/2
  Sum1/1 -> Product2/2
  Temperature Standard/1 -> Sum1/2
  Temp/1 -> Sum2/1
  Sum2/1 -> Sum1/1
  Product3/1 -> Sum2/2
  NOCT - 20/1 -> Product3/1
  Divide/1 -> Product3/2
  W/m/1 -> Divide/2
  Ir/1 -> Divide/1, Product/3
  Constant1/1 -> Max/2
  Max/1 -> PowerOut/1
  Product1/1 -> Max/1

== system FullyConnectedMMG/Subsystem1/Microgrid 2/Active Power Dynamics ==
  In : Inport
  1/Tp : Gain  Gain=1/0.004
  Integrator : Integrator
  Sum : Sum  Inputs=|+-
  Out : Outport  VectorParamsAs1DForOutWhenUnconnected=off
  wires:
  Sum/1 -> 1/Tp/1
  1/Tp/1 -> Integrator/1
  In/1 -> Sum/1
  Integrator/1 -> Sum/2, Out/1

== system FullyConnectedMMG/Subsystem1/Microgrid 2/Energy Storage ==
  Pref : Inport
  Qref : Inport  Port=2
  Charge Limits : Subsystem
  Mux1 : Mux  Inputs=2
  Power Limits : Saturate  UpperLimit=Pnom  LowerLimit=-Pnom
  Reactive Power Capability : Subsystem
  Simple Battery Inverter : powerlib/Elements/Three-Phase Dynamic Load  NominalVoltage=[Vn Fn]  ActiveReactivePowers=[-500000 -3.38813e-13]  PositiveSequence=[0.999844 -0.0038635]  ExternalControl=on  NpNq=[1.3 2]  TimeConstants="[0  0  0  0]"  MinimumVoltage=0.7  Tfilter=1e-2  LoadFlowParameters=[4,0,0,0,0]
      link override Model/Discrete 3-phase PLL: Ts=Ts
      link override Model/Discrete 3-phase PLL/Discrete PI Controller: Ts=Ts
      link override Model/Discrete 3-phase PLL/Discrete Rate Limiter: Ts=Ts
      link override Model/Discrete 3-phase PLL/Discrete Variable Frequency Mean value: Ts=Ts
      link override Model/Discrete 3-phase PLL/Discrete  2nd-Order Filter: Ts=Ts
      link override Model/Mean (Variable Frequency): Ts=Ts
      link override Model/Mean (Variable Frequency)1: Ts=Ts
      settings: SourceProductBaseCode=PS
  Stored Energy Calculation (%) : Subsystem
  Terminator : Terminator
  Unary Minus : UnaryMinus
  A : PMIOPort  Side=Right
  B : PMIOPort  Port=2  Side=Right
  C : PMIOPort  Port=3  Side=Right
  SOC (%) : Outport  VectorParamsAs1DForOutWhenUnconnected=off
  Pbatt : Outport  Port=2  VectorParamsAs1DForOutWhenUnconnected=off
  wires:
  Charge Limits/2(Qbatt) -> Reactive Power Capability/2(Qin)
  Qref/1 -> Charge Limits/3(Qin)
  Power Limits/1 -> Charge Limits/2(Pin)
  Charge Limits/1(Pbatt) -> Reactive Power Capability/1(Pin), Unary Minus/1, Pbatt/1, Stored Energy Calculation (%)/1(Pin)  "Pbatt"
  Stored Energy Calculation (%)/1(SE%) -> SOC (%)/1, Charge Limits/1(SOC (%))  "SOC (%)"
  Pref/1 -> Power Limits/1
  Reactive Power Capability/1(Qout) -> Mux1/2, Stored Energy Calculation (%)/2(Qin)  "Qbatt"
  Simple Battery Inverter/1 -> Terminator/1
  Mux1/1 -> Simple Battery Inverter/1
  Unary Minus/1 -> Mux1/1
  connections:
  Simple Battery Inverter/LConn1 -- A/RConn1
  Simple Battery Inverter/LConn3 -- C/RConn1
  Simple Battery Inverter/LConn2 -- B/RConn1

== system FullyConnectedMMG/Subsystem1/Microgrid 2/Power Equation Wind Turbine (PQ Model)1 ==
  Wind (m/s) : Inport
  Qref (pu) : Inport  Port=2
  Active Power Dynamics : Subsystem  VariantControl=T6NotZero
      mask Display: disp('1 / (1 + s T_P)','texmode','on');
  Ground : powerlib/Elements/Ground  LConnTagsString=a
  Mux : Mux  Inputs=2
  Reactive Power Dynamics : Subsystem  VariantControl=T6NotZero
      mask Display: disp('1 / (1 + s T_Q)','texmode','on');
  Saturation : Saturate  UpperLimit=Qmax  LowerLimit=-Qmax
  Shunt (Numerical Stability) : powerlib/Elements/Three-Phase Series RLC Branch  LConnTagsString=A|B|C  RConnTagsString=A|B|C  BranchType=R  Resistance=1e9  Inductance=1e-3  Capacitance=1e-6  Measurements=None
  Three-Phase Dynamic Load : powerlib/Elements/Three-Phase Dynamic Load  NominalVoltage=[575 60]  ActiveReactivePowers=[20e3 1e3]  PositiveSequence=[0.994 -11.8]  ExternalControl=on  NpNq=[1.3 2]  TimeConstants="[0  0  0  0]"  MinimumVoltage=0.7  Tfilter=1e-4  LoadFlowParameters=[4,0,0,0,0]
      link override Model/Discrete 3-phase PLL: Ts=Ts
      link override Model/Discrete 3-phase PLL/Discrete PI Controller: Ts=Ts
      link override Model/Discrete 3-phase PLL/Discrete Rate Limiter: Ts=Ts
      link override Model/Discrete 3-phase PLL/Discrete Variable Frequency Mean value: Ts=Ts
      link override Model/Discrete 3-phase PLL/Discrete  2nd-Order Filter: Ts=Ts
      link override Model/Mean (Variable Frequency): Ts=Ts
      link override Model/Mean (Variable Frequency)1: Ts=Ts
      settings: SourceProductBaseCode=PS
  Unary Minus : UnaryMinus
  Wind Turbine Power Equation : Subsystem
  A : PMIOPort  Side=Left
  B : PMIOPort  Port=2  Side=Left
  C : PMIOPort  Port=3  Side=Left
  m : Outport  VectorParamsAs1DForOutWhenUnconnected=off
  wires:
  Qref (pu)/1 -> Saturation/1
  Saturation/1 -> Reactive Power Dynamics/1(In)
  Reactive Power Dynamics/1(Out) -> Mux/2
  Mux/1 -> Three-Phase Dynamic Load/1
  Wind (m/s)/1 -> Wind Turbine Power Equation/1(Wind (m/s))
  Three-Phase Dynamic Load/1 -> m/1
  Wind Turbine Power Equation/1(Pwind) -> Active Power Dynamics/1(In)
  Active Power Dynamics/1(Out) -> Unary Minus/1
  Unary Minus/1 -> Mux/1
  connections:
  Ground/LConn1 -- Shunt (Numerical Stability)/RConn1 -- Shunt (Numerical Stability)/RConn2 -- Shunt (Numerical Stability)/RConn3
  Shunt (Numerical Stability)/LConn1 -- Three-Phase Dynamic Load/LConn1 -- A/RConn1
  Shunt (Numerical Stability)/LConn3 -- Three-Phase Dynamic Load/LConn3 -- C/RConn1
  Shunt (Numerical Stability)/LConn2 -- Three-Phase Dynamic Load/LConn2 -- B/RConn1

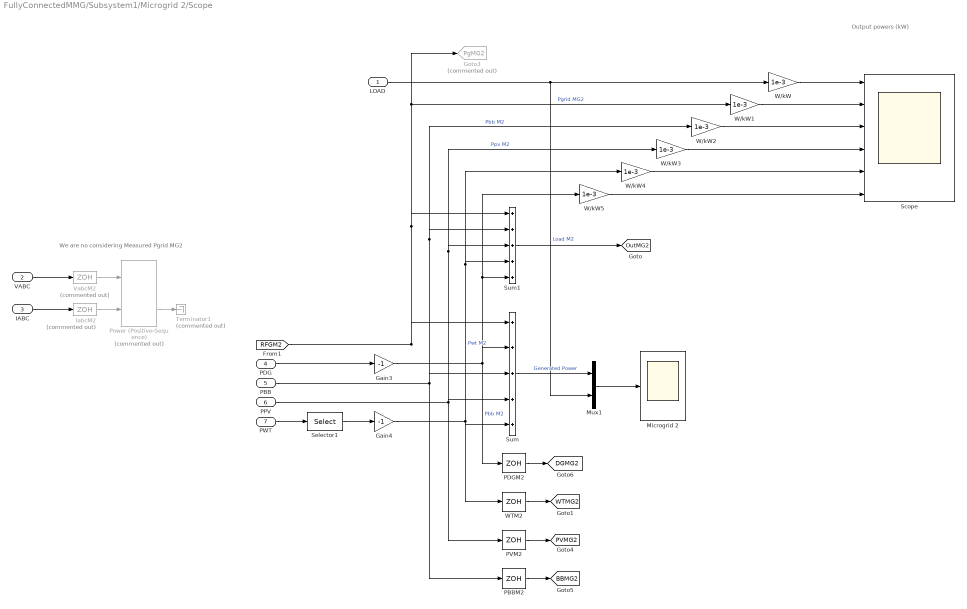
== system FullyConnectedMMG/Subsystem1/Microgrid 2/Scope ==
  note: We are no considering Measured Pgrid MG2
  note: Output powers (kW)
  LOAD : Inport
  VABC : Inport  Port=2
  IABC : Inport  Port=3
  PDG : Inport  Port=4
  PBB : Inport  Port=5
  PPV : Inport  Port=6
  PWT : Inport  Port=7
  Gain3 : Gain  Gain=-1
  Gain4 : Gain  Gain=-1
  Goto3 : Goto  Commented=on  GotoTag=PgMG2  TagVisibility=global
  IabcM2 : ZeroOrderHold  Commented=on  SampleTime=Ts
  Microgrid 2 : Scope
  Mux1 : Mux  Inputs=2
  PBBM2 : ZeroOrderHold  SampleTime=Ts
  PDGM2 : ZeroOrderHold  SampleTime=Ts
  PVM2 : ZeroOrderHold  SampleTime=Ts
  Power (Positive-Sequence) : powerlib_meascontrol/Measurements/Power (Positive-Sequence)  Commented=on  Freq=60  Vinit=[0, 0]  Iinit=[0, 0]  Ts=3e-4
      settings: SourceProductBaseCode=PS
  Scope : Scope  NumInputPorts=6
  Selector1 : Selector  InputPortWidth=3  IndexOptions=Index vector (dialog)  Indices=[2]  OutputSizes=1
  Sum : Sum  Inputs=|+++++
  Sum1 : Sum  Inputs=|+++++
  Terminator1 : Terminator  Commented=on
  VabcM2 : ZeroOrderHold  Commented=on  SampleTime=Ts
  W/kW{,1..5} (6 alike) : Gain  Gain=1e-3
  WTM2 : ZeroOrderHold  SampleTime=Ts
  tag scope: BBMG2=global, DGMG2=global, OutMG2=global, PVMG2=global, WTMG2=global
  wires:
  Selector1/1 -> Gain4/1
  PWT/1 -> Selector1/1
  Gain4/1 -> Sum/5, WTM2/1, Sum1/4, W/kW4/1  "Pwt M2"
  LOAD/1 -> Mux1/2, W/kW/1  "Load M2"
  Mux1/1 -> Microgrid 2/1
  Sum/1 -> Mux1/1  "Generated Power"
  [RFGM2] -> Sum1/1, Goto3/1, W/kW1/1, Sum/1  "Pgrid MG2"
  PBB/1 -> PBBM2/1, Sum/3, W/kW2/1, Sum1/2  "Pbb M2"
  PPV/1 -> PVM2/1, Sum/4, Sum1/3, W/kW3/1  "Ppv M2"
  Power (Positive-Sequence)/2 -> Terminator1/1
  VABC/1 -> VabcM2/1
  Sum1/1 -> [OutMG2]
  PDG/1 -> Gain3/1
  Gain3/1 -> PDGM2/1, Sum/2, Sum1/5, W/kW5/1  "Pbb M2"
  PDGM2/1 -> [DGMG2]
  PBBM2/1 -> [BBMG2]
  PVM2/1 -> [PVMG2]
  WTM2/1 -> [WTMG2]
  VabcM2/1 -> Power (Positive-Sequence)/1
  IabcM2/1 -> Power (Positive-Sequence)/2
  IABC/1 -> IabcM2/1
  W/kW/1 -> Scope/1
  W/kW1/1 -> Scope/2
  W/kW2/1 -> Scope/3
  W/kW3/1 -> Scope/4
  W/kW4/1 -> Scope/5
  W/kW5/1 -> Scope/6

== system FullyConnectedMMG/Subsystem1/Microgrid 2/Simple Diesel Generator ==
  Pref (pu) : Inport
  Qref (pu) : Inport  Port=2
  Active Power Dynamics : Subsystem  VariantControl=T6NotZero
      mask Display: disp('1 / (1 + s T_P)','texmode','on');
  Ground : powerlib/Elements/Ground  LConnTagsString=a
  Mux : Mux  Inputs=2
  Reactive Power Dynamics : Subsystem  VariantControl=T6NotZero
      mask Display: disp('1 / (1 + s T_Q)','texmode','on');
  Saturation : Saturate  UpperLimit=Qmax  LowerLimit=-Qmax
  Shunt (Numerical Stability) : powerlib/Elements/Three-Phase Series RLC Branch  LConnTagsString=A|B|C  RConnTagsString=A|B|C  BranchType=R  Resistance=1e3  Inductance=1e-3  Capacitance=1e-6  Measurements=None
  Three-Phase Dynamic Load : powerlib/Elements/Three-Phase Dynamic Load  NominalVoltage=[Vn Fn]  ActiveReactivePowers=[20e3 1e3]  PositiveSequence=[0.994 -11.8]  ExternalControl=on  NpNq=[1.3 2]  TimeConstants="[0  0  0  0]"  MinimumVoltage=0.7  Tfilter=1e-4  LoadFlowParameters=[4,0,0,0,0]
      link override Model/Discrete 3-phase PLL: Ts=Ts
      link override Model/Discrete 3-phase PLL/Discrete PI Controller: Ts=Ts
      link override Model/Discrete 3-phase PLL/Discrete Rate Limiter: Ts=Ts
      link override Model/Discrete 3-phase PLL/Discrete Variable Frequency Mean value: Ts=Ts
      link override Model/Discrete 3-phase PLL/Discrete  2nd-Order Filter: Ts=Ts
      link override Model/Mean (Variable Frequency): Ts=Ts
      link override Model/Mean (Variable Frequency)1: Ts=Ts
      settings: SourceProductBaseCode=PS
  Unary Minus : UnaryMinus
  A : PMIOPort  Side=Left
  B : PMIOPort  Port=2  Side=Left
  C : PMIOPort  Port=3  Side=Left
  m : Outport  VectorParamsAs1DForOutWhenUnconnected=off
  wires:
  Pref (pu)/1 -> Active Power Dynamics/1(In)
  Mux/1 -> Three-Phase Dynamic Load/1
  Reactive Power Dynamics/1(Out) -> Mux/2
  Saturation/1 -> Reactive Power Dynamics/1(In)
  Qref (pu)/1 -> Saturation/1
  Three-Phase Dynamic Load/1 -> m/1
  Active Power Dynamics/1(Out) -> Unary Minus/1
  Unary Minus/1 -> Mux/1
  connections:
  B/RConn1 -- Shunt (Numerical Stability)/LConn2 -- Three-Phase Dynamic Load/LConn2
  C/RConn1 -- Shunt (Numerical Stability)/LConn3 -- Three-Phase Dynamic Load/LConn3
  A/RConn1 -- Shunt (Numerical Stability)/LConn1 -- Three-Phase Dynamic Load/LConn1
  Shunt (Numerical Stability)/RConn3 -- Shunt (Numerical Stability)/RConn2 -- Shunt (Numerical Stability)/RConn1 -- Ground/LConn1

== system FullyConnectedMMG/Subsystem1/Microgrid 2/Solar Array ==
  P : Inport
  Active Power Dynamics : Subsystem  VariantControl=T6NotZero
      mask Display: disp('1 / (1 + s T_P)','texmode','on');
  Bus Selector : BusSelector  OutputSignals=Active power P (W)
  Constant11 : Constant  Value=0
  Mux1 : Mux  Inputs=2
  Simple Solar Inverter : powerlib/Elements/Three-Phase Dynamic Load  NominalVoltage=[Vn Fn]  ActiveReactivePowers=[-250000 -3.38813e-13]  PositiveSequence=[0.999844 -0.0038635]  ExternalControl=on  NpNq=[1.3 2]  TimeConstants="[0  0  0  0]"  MinimumVoltage=0.7  Tfilter=1e-2  LoadFlowParameters=[4,0,0,0,0]
      link override Model/Discrete 3-phase PLL: Ts=Ts
      link override Model/Discrete 3-phase PLL/Discrete PI Controller: Ts=Ts
      link override Model/Discrete 3-phase PLL/Discrete Rate Limiter: Ts=Ts
      link override Model/Discrete 3-phase PLL/Discrete Variable Frequency Mean value: Ts=Ts
      link override Model/Discrete 3-phase PLL/Discrete  2nd-Order Filter: Ts=Ts
      link override Model/Mean (Variable Frequency): Ts=Ts
      link override Model/Mean (Variable Frequency)1: Ts=Ts
      settings: SourceProductBaseCode=PS
  Unary Minus : UnaryMinus
  Unary Minus1 : UnaryMinus
  A : PMIOPort  Side=Right
  B : PMIOPort  Port=2  Side=Right
  C : PMIOPort  Port=3  Side=Right
  m : Outport  VectorParamsAs1DForOutWhenUnconnected=off
  wires:
  Unary Minus1/1 -> m/1
  Bus Selector/1 -> Unary Minus1/1  "<Active power P (W)>"
  Simple Solar Inverter/1 -> Bus Selector/1
  Constant11/1 -> Mux1/2
  Mux1/1 -> Simple Solar Inverter/1
  Unary Minus/1 -> Mux1/1
  P/1 -> Active Power Dynamics/1(In)
  Active Power Dynamics/1(Out) -> Unary Minus/1
  connections:
  Simple Solar Inverter/LConn1 -- A/RConn1
  Simple Solar Inverter/LConn3 -- C/RConn1
  Simple Solar Inverter/LConn2 -- B/RConn1

== system FullyConnectedMMG/Subsystem1/Microgrid 2/Variable Load ==
  Load : Inport
  Active Power Dynamics : Subsystem  VariantControl=T6NotZero
      mask Display: disp('1 / (1 + s T_P)','texmode','on');
  Dynamic Load Control : Subsystem
  Simple Three-Phase Load : powerlib/Elements/Three-Phase Dynamic Load  NominalVoltage=[Vn Fn]  ActiveReactivePowers=[200000 45883.1]  PositiveSequence=[0.999844 -0.0038635]  ExternalControl=on  NpNq=[1.3 2]  TimeConstants="[0  0  0  0]"  MinimumVoltage=0.7  Tfilter=1e-2  LoadFlowParameters=[4,0,0,0,0]
      link override Model/Discrete 3-phase PLL: Ts=Ts
      link override Model/Discrete 3-phase PLL/Discrete PI Controller: Ts=Ts
      link override Model/Discrete 3-phase PLL/Discrete Rate Limiter: Ts=Ts
      link override Model/Discrete 3-phase PLL/Discrete Variable Frequency Mean value: Ts=Ts
      link override Model/Discrete 3-phase PLL/Discrete  2nd-Order Filter: Ts=Ts
      link override Model/Mean (Variable Frequency): Ts=Ts
      link override Model/Mean (Variable Frequency)1: Ts=Ts
      settings: SourceProductBaseCode=PS
  Terminator : Terminator
  A : PMIOPort  Side=Right
  B : PMIOPort  Port=2  Side=Right
  C : PMIOPort  Port=3  Side=Right
  wires:
  Dynamic Load Control/1(PQ) -> Simple Three-Phase Load/1
  Load/1 -> Active Power Dynamics/1(In)
  Simple Three-Phase Load/1 -> Terminator/1
  Active Power Dynamics/1(Out) -> Dynamic Load Control/1(P0)
  connections:
  Simple Three-Phase Load/LConn2 -- B/RConn1
  Simple Three-Phase Load/LConn3 -- C/RConn1
  Simple Three-Phase Load/LConn1 -- A/RConn1
